simulink model "VZXA_DFPM_SA_MdlIdent"  (R2017a)
settings: Solver=VariableStepAuto  StartTime=0.0  StopTime=70  FixedStep=0.00005  MaxStep=.005  RelTol=1e-5  EnableMultiTasking=on
undefined symbols (not defined in the file or in its folder): mdlPara
libraries: PASL_Models x1, PASL_Tools x1
settings Model: Creator=fbwk  LastModifiedBy=mmnt
settings SolverCC: SolverResetMethod=Robust
settings DataIOCC: LimitDataPoints=on  SaveFormat=Array  SaveOutput=off  SignalLogging=off  DSMLogging=off  SaveTime=off
settings OptimizationCC: LifeSpan=inf
settings DebuggingCC: SolverPrmCheckMsg=warning  SFUnexpectedBacktrackingDiag=warning  SFNoUnconditionalDefaultTransitionDiag=warning  SFExecutionAtInitializationDiag=none
settings HardwareCC: ProdBitPerPointer=32  ProdBitPerSizeT=32  ProdBitPerPtrDiffT=32  ProdLargestAtomicFloat=None  ProdIntDivRoundTo=Undefined  ProdEndianess=Unspecified  ProdWordSize=32  ProdHWDeviceType=32-bit Generic
settings ModelReferenceCC: PropagateSignalLabelsOutOfModel=off
settings GRTTargetCC: TargetLangStandard=C89/C90 (ANSI)  GeneratePreprocessorConditionals=Disable all
settings ConfigComp: CovMetricSettings=dw  CovHtmlReporting=on  CovSaveCumulativeToWorkspaceVar=on  CovSaveSingleToWorkspaceVar=on  CovExternalEMLEnable=off  CovSFcnEnable=off

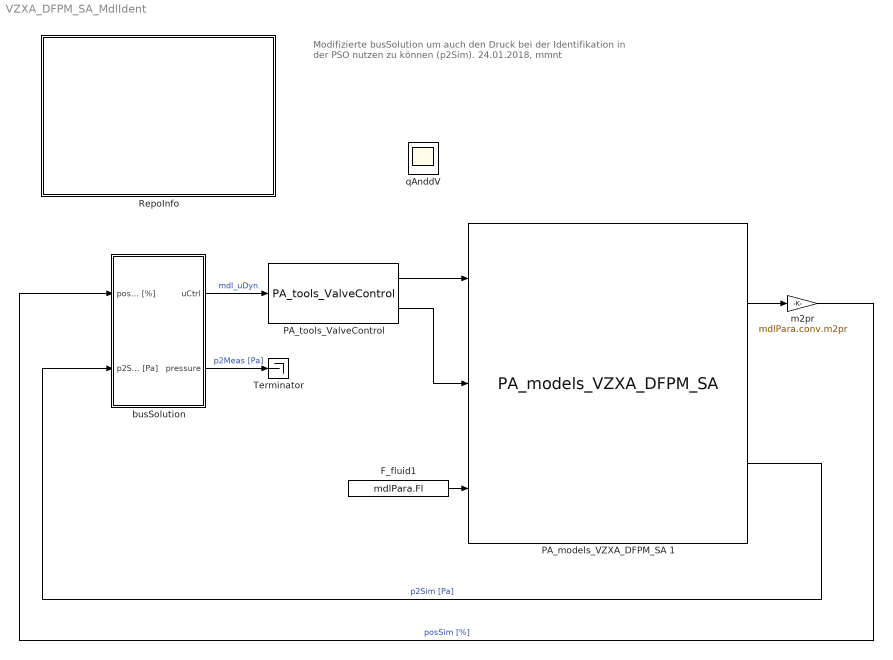
== system VZXA_DFPM_SA_MdlIdent ==
  note: Modifizierte busSolution um auch den Druck bei der Identifikation
      | in der PSO nutzen zu können (p2Sim).
      | 24.01.2018, mmnt
  F_fluid1 : Constant  Value=mdlPara.Fl
  PA_models_VZXA_DFPM_SA 1 : PASL_Models/PA_models_VZXA_DFPM_SA   Tag=PA_models_CMSI_piston_singleActing  mdlPara=mdlPara
      settings: SourceProductName=PASL
  PA_tools_ValveControl : PASL_Tools/PA_tools_ValveControl
      settings: SourceProductName=PASL
  RepoInfo : Subsystem  Tag=RevTagSubSys  AncestorBlock=PASL_Tools/RepoInfo  mask(cover){}
      mask help: mask for library reasons
      settings: OpenFcn=PA_setRepoInfoBlock()
      mask Display: text(.05,.95,'Project:\n   Rev#:  32\n   RevID: 8225ca25589b\n   date:  Wed Jan 17 08:22:27 2018 +0100\n\nPASL:\n   Rev#:  450\n   RevID: daf3a9f880be\n   date:  Mon Jan 22 09:15:51 2018 +0100\n\nPATL:\n   Rev#:  69\n   RevID: 4f4fb19223fd\n   date:  Mon Jan 22 16:50:01 2018 +0100','hor','left','ver','top')
  Terminator : Terminator
  busSolution : Subsystem  VariantControl=busVariant
  m2pr : Gain  Gain=mdlPara.conv.m2pr  OutDataTypeStr=single
  qAnddV : Scope
  wires:
  m2pr/1 -> busSolution/1(posSim [%])  "posSim [%]"
  busSolution/1(uCtrl) -> PA_tools_ValveControl/1  "mdl_uDyn"
  PA_models_VZXA_DFPM_SA 1/2 -> busSolution/2(p2Sim [Pa])  "p2Sim [Pa]"
  PA_tools_ValveControl/1 -> PA_models_VZXA_DFPM_SA 1/1
  PA_tools_ValveControl/2 -> PA_models_VZXA_DFPM_SA 1/2
  busSolution/2(pressure) -> Terminator/1  "p2Meas [Pa]"
  PA_models_VZXA_DFPM_SA 1/1 -> m2pr/1
  F_fluid1/1 -> PA_models_VZXA_DFPM_SA 1/3

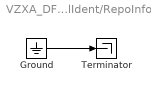
== system VZXA_DFPM_SA_MdlIdent/RepoInfo ==
  Ground : Ground
  Terminator : Terminator
  wires:
  Ground/1 -> Terminator/1

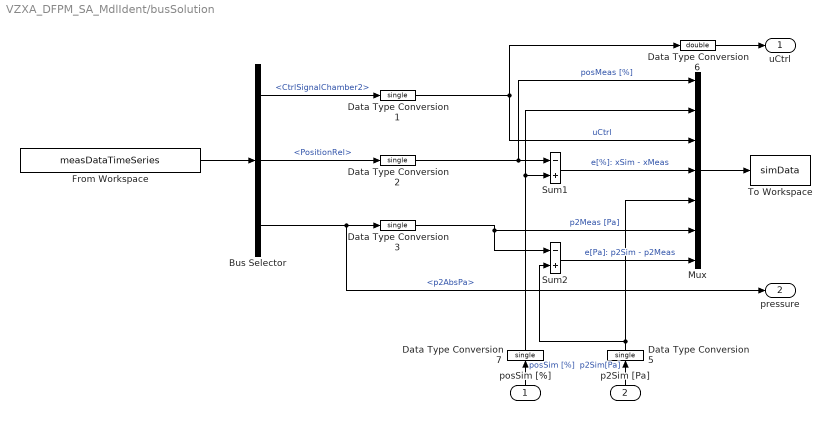
== system VZXA_DFPM_SA_MdlIdent/busSolution ==
  posSim [%] : Inport
  p2Sim [Pa] : Inport  Port=2
  Bus Selector : BusSelector  OutputSignals=CtrlSignalChamber2,PositionRel,p2AbsPa
  Data Type Conversion{1..3,5,7} (5 alike) : DataTypeConversion  OutDataTypeStr=single
  Data Type Conversion6 : DataTypeConversion  OutDataTypeStr=double
  From Workspace : FromWorkspace  VariableName=measDataTimeSeries  OutDataTypeStr=Bus: busMeasData  SampleTime=0
  Mux : Mux  Inputs=7
  Sum1 : Sum  Inputs=-+
  Sum2 : Sum  Inputs=-+
  To Workspace : ToWorkspace  VariableName=simData  SaveFormat=Structure With Time  SampleTime=-1
  uCtrl : Outport
  pressure : Outport  Port=2
  wires:
  Bus Selector/3 -> pressure/1, Data Type Conversion3/1  "<p2AbsPa>"
  Bus Selector/1 -> Data Type Conversion1/1  "<CtrlSignalChamber2>"
  From Workspace/1 -> Bus Selector/1
  Bus Selector/2 -> Data Type Conversion2/1  "<PositionRel>"
  posSim [%]/1 -> Data Type Conversion7/1  "posSim [%]"
  Sum1/1 -> Mux/4  "e[%]: xSim - xMeas"
  Mux/1 -> To Workspace/1
  Data Type Conversion1/1 -> Mux/3, Data Type Conversion6/1  "uCtrl"
  Data Type Conversion2/1 -> Sum1/1, Mux/1  "posMeas [%]"
  Data Type Conversion3/1 -> Sum2/1, Mux/6  "p2Meas [Pa]"
  p2Sim [Pa]/1 -> Data Type Conversion5/1  "p2Sim[Pa]"
  Sum2/1 -> Mux/7  "e[Pa]: p2Sim - p2Meas"
  Data Type Conversion6/1 -> uCtrl/1
  Data Type Conversion7/1 -> Mux/2, Sum1/2
  Data Type Conversion5/1 -> Mux/5, Sum2/2
